simulink model "flightControlSystem"  (R2021a)
settings: Solver=ode3  StartTime=0  StopTime=TFinal  FixedStep=Ts  RelTol=1e-3  EnableMultiTasking=on
model workspace (MAT data in the model file):
  circlePoints = [9575 9695 9815 9935 10055 10175 10295 10294 10414 10534 10654 10774 ... (270 elements, 1x270)]
  rad = [-3.14159265359 -3.12159265359 -3.09159265359 -3.06159265359 -3.03159265359 -3.01159265359 -2.98159265359 -2.97159265359 -2.95159265359 -2.92159265359 -2.89159265359 -2.86159265359 ... (270 elements, 1x270)]
undefined symbols (not defined in the file): codertarget, Controller, DiscIntNeverNeededParam, Discrete, Estimator, g, gray, init, Sensors, Time, Ts, var_acc_angle_N, var_bias_gyr_N, var_gyro_p_N, Vehicle
libraries: simulink x41, pid_lib x4, ctrlSharedLib x4, sharedtransform x3, fuzblock x1, visionstatistics x1, visiontextngfix x1, parrotlib x1
(part 3 of 3)

== matlab function flightControlSystem/Control System/Path Planning/Flight State Flow/Flight/MATLAB Function1 ==
  data: majorDirection input; Direction input; maskedPoints output; movingSideRatio output; limDirection output; corner output; Points input; rad input
function [maskedPoints,movingSideRatio,limDirection,corner] = fcn(majorDirection,Direction,Points,rad)
persistent detectCorner ts
if isempty(detectCorner)
	detectCorner = false;
	ts = 5;
end
movingSideRatio = 0;
limDirection1 = 0;
limDirection2 = 0;
if ~isnan(Direction)
	if detectCorner
		radwidth = deg2rad(30);
		limDirection1 = majorDirection+radwidth/2;
		limDirection2 = majorDirection-radwidth/2;
	else
		radwidth = deg2rad(45);
		limDirection1 = Direction+radwidth/2;
		limDirection2 = Direction-radwidth/2;
	end
    if pi < limDirection1
        limDirection1 = limDirection1-2*pi;
    end
    if -pi > limDirection2
        limDirection2 = limDirection2+2*pi;
    end
    if limDirection1-limDirection2 > 0
        indexlist = rad(1,:)<limDirection1 & rad(1,:)>limDirection2;
    else
        indexlist = rad(1,:)<limDirection1 | rad(1,:)>limDirection2;
    end
    movingSideRatio = length(find(Points(1,indexlist)))/length(Points(1,indexlist));
	if movingSideRatio == 1
		detectCorner = true;
	end

	if movingSideRatio == 0 && detectCorner && ~isnan(majorDirection)
        ignore_width = deg2rad(40);
        oppoSide = majorDirection+pi;
		detectCorner = false;
		ts = 0;
	elseif (detectCorner) && ~isnan(majorDirection)
		ignore_width = deg2rad(340);
		oppoSide = majorDirection+pi;
	else
		if ts < 4; ts=ts+0.005; end
		bias = -0.0065*ts^2 + 1.06;
		if bias<1; bias=1; end
        ignore_width = 5.2 * bias;
		oppoSide = Direction+pi;
	end
	if oppoSide > pi
		oppoSide = oppoSide-2*pi;
	end
    limDirection1 = oppoSide+ignore_width/2;
    limDirection2 = oppoSide-ignore_width/2;
    if pi < limDirection1
        limDirection1 = limDirection1-2*pi;
    end
    if -pi > limDirection2
        limDirection2 = limDirection2+2*pi;
    end
    if limDirection1-limDirection2 > 0
        indexlist = rad(1,:)<limDirection1 & rad(1,:)>limDirection2;
    else
        indexlist = rad(1,:)<limDirection1 | rad(1,:)>limDirection2;
    end
    Points(1,indexlist) = 0;
end
corner = detectCorner;
maskedPoints = [Points;rad];
limDirection = [limDirection1;limDirection2];
